simulink model "prob_3"  (R2020b)
settings: Solver=VariableStepAuto  StartTime=0.0  StopTime=10.0  RelTol=1e-3
settings Model: Creator=Akshay A H  LastModifiedBy=Akshay A H

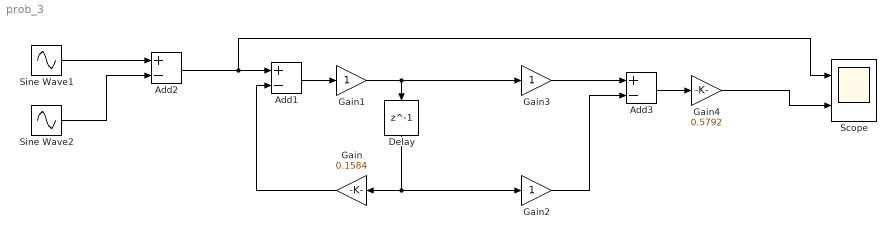
== system prob_3 ==
  Add1 : Sum  Inputs=+-
  Add2 : Sum  Inputs=+-
  Add3 : Sum  Inputs=+-
  Delay : Delay  DelayLength=1
  Gain : Gain  Gain=0.1584
  Gain1 : Gain
  Gain2 : Gain
  Gain3 : Gain
  Gain4 : Gain  Gain=0.5792
  Scope : Scope  NumInputPorts=2
  Sine Wave1 : Sin  SampleTime=0
  Sine Wave2 : Sin  Amplitude=0.00001  Frequency=7500  SampleTime=0
  wires:
  Gain/1 -> Add1/2
  Sine Wave2/1 -> Add2/2
  Add3/1 -> Gain4/1
  Gain2/1 -> Add3/2
  Gain3/1 -> Add3/1
  Add2/1 -> Scope/1, Add1/1
  Gain1/1 -> Gain3/1, Delay/1
  Add1/1 -> Gain1/1
  Delay/1 -> Gain2/1, Gain/1
  Sine Wave1/1 -> Add2/1
  Gain4/1 -> Scope/2
